simulink model "Model0"  (R2022b)
settings: Solver=VariableStepAuto  StartTime=0.0  StopTime=10.0  RelTol=1e-3
undefined symbols (not defined in the file or in its folder): commpassbandmodParams, qam_params
libraries: hdlsllib x14, dspsrcs4 x9, commfilt2 x8, commdigbbndam3 x8
settings Model: Creator=Ceribro  LastModifiedBy=Ceribro

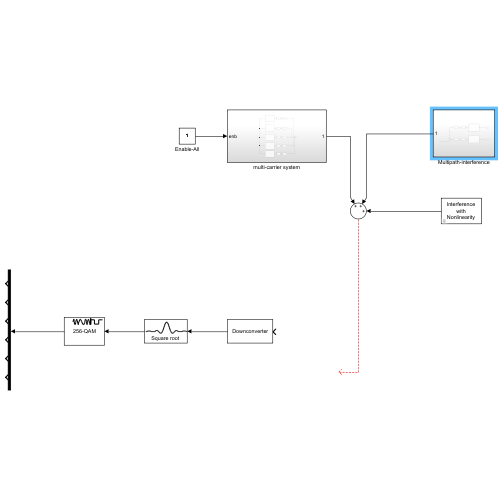
[thumbnail: Simulink's stored preview of the top-level diagram]
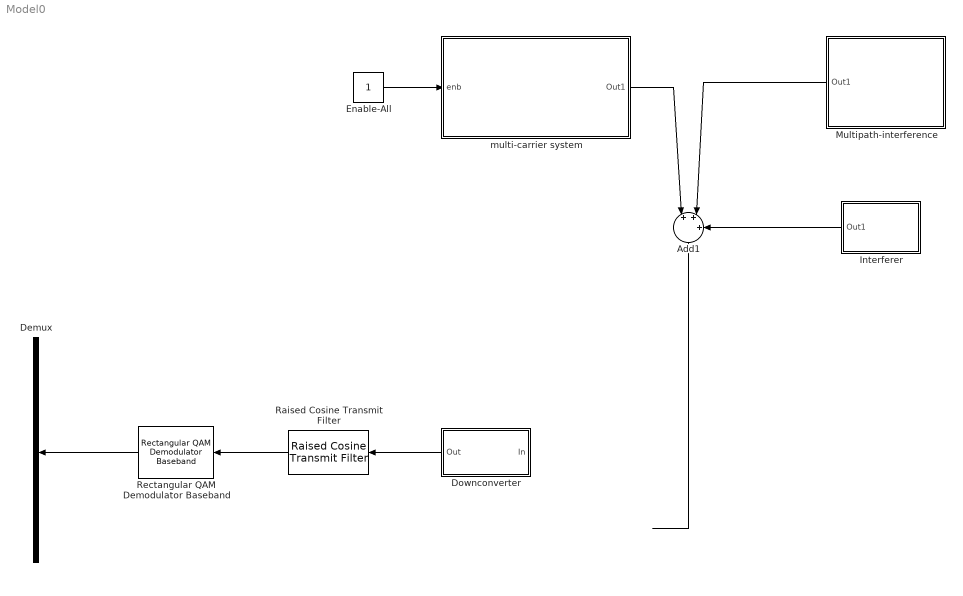
== system Model0 ==
  Add1 : Sum  Inputs=|+++
  Demux : Demux  Outputs=6
  Downconverter : Subsystem
      mask Display: disp('Downconverter')
  Enable-All : Constant  OutDataTypeStr=boolean
  Interferer : Subsystem  mask(Interference){nonlinOrder=3}
      mask prompts: nonlinOrder "Order of nonlinearity:"
      mask help: Generate out-of-band interference. Optionally process the interference with a third-order nonlinearity that creates an in-band harmonic.
      mask init:
      | if nonlinOrder == 1
      |     icontext = 'Interference\nwithout\nNonlinearity';
      | elseif nonlinOrder == 3
      |     icontext = 'Interference\nwith\nNonlinearity';
      | end
      mask Display: disp(icontext)
  Multipath-interference : Subsystem
  Raised Cosine Transmit Filter : commfilt2/Raised Cosine Transmit Filter  filtType=Square root  R=0.2  filtSpan=8  N=8  filterGain=1  InputProcessing=Columns as channels (frame based)  RateOptions=Enforce single-rate processing  framing=Mute  checkCoeff=off  variableName=rcTxFilt1  checkGain=Normalized  sampMode=Mute  saveAsFlag=0  currentFiltSpan=2*(4)  D=4  launchFVT=off  roundingMode=Floor  overflowMode=off  coeffDataTypeStr=Inherit: Same word length as input  coeffMin=[]  coeffMax=[]  coeffLastDataTypeStr=Inherit: Same word length as input  outputDataTypeStr=Inherit: Same as accumulator  outputMin=[]  outputMax=[]  outputLastDataTypeStr=Inherit: Same as accumulator
  Rectangular QAM Demodulator Baseband : commdigbbndam3/Rectangular QAM Demodulator Baseband  M=256  OutType=Integer  DecType=Hard decision  VarSource=Dialog  Variance=1  Dec=Gray  Mapping=[0:15]  PowType=Min. distance between symbols  MinDist=2  AvgPow=1  PeakPow=1  Ph=0  outDtype1=Inherit via internal rule  outDtype2=Inherit via internal rule  derotateFactorWordLen=16  derotateFactorDataTypeStr=Inherit: Same word length as input  derotateFactorLastDataTypeStr=Inherit: Same word length as input  denormFactorWordLen=16  denormFactorDataTypeStr=Inherit: Same word length as input  denormFactorLastDataTypeStr=Inherit: Same word length as input  prodOutWordLen=32  prodOutOverflowMode=Wrap  prodOutRoundingMode=Floor  prodOutOvFlMode=off  prodOutOvFlModeLastStrValue=off  sumWordLen=32
      settings: LibrarySourceBlock=|
      | commhdldigbbndam/Rectangular QAM
      | Demodulator
      | Baseband
  multi-carrier system : Subsystem
  wires:
  Enable-All/1 -> multi-carrier system/1(enb)
  multi-carrier system/1(Out1) -> Add1/1
  Multipath-interference/1(Out1) -> Add1/2
  Interferer/1(Out1) -> Add1/3
  Add1/1 -> ?
  Downconverter/1(Out) -> Raised Cosine Transmit Filter/1
  Raised Cosine Transmit Filter/1 -> Rectangular QAM Demodulator Baseband/1
  Rectangular QAM Demodulator Baseband/1 -> Demux/1

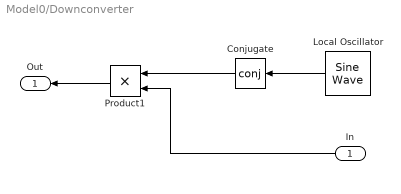
== system Model0/Downconverter ==
  In : Inport
  Conjugate : Math  Operator=conj  SignedPower=on
  Local Oscillator : dspsrcs4/Sine Wave  Amplitude=1  Frequency=commpassbandmodParams.Fc  Phase=0  SampleMode=Discrete  OutComplex=Complex  CompMethod=Trigonometric fcn  TableSize=Speed  SampleTime=(1e-6) /8  SamplesPerFrame=800  ResetState=Restart at time zero  OutputFrames=off  dataType=double  wordLen=16  udDataType=sfix(16)  fracBitsMode=Best precision  numFracBits=15  OutDataTypeStr=double  LastOutDataTypeStr=double
  Product1 : Product  RndMeth=Zero
  Out : Outport  VectorParamsAs1DForOutWhenUnconnected=off
  wires:
  Conjugate/1 -> Product1/1
  Product1/1 -> Out/1
  In/1 -> Product1/2
  Local Oscillator/1 -> Conjugate/1

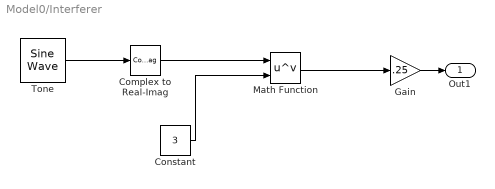
== system Model0/Interferer ==
  Complex to Real-Imag : ComplexToRealImag  Output=Real
  Constant : Constant  Value=3
  Gain : Gain  Gain=.25
  Math Function : Math  Operator=pow  SignedPower=on
  "Tone " : dspsrcs4/Sine Wave  Amplitude=1  Frequency=8.8333e+05  Phase=0  SampleMode=Discrete  OutComplex=Complex  CompMethod=Trigonometric fcn  TableSize=Speed  SampleTime=(1e-6) /8  SamplesPerFrame=800  ResetState=Restart at time zero  OutputFrames=off  dataType=double  wordLen=16  udDataType=sfix(16)  fracBitsMode=Best precision  numFracBits=15  OutDataTypeStr=double  LastOutDataTypeStr=double
  Out1 : Outport  VectorParamsAs1DForOutWhenUnconnected=off
  wires:
  Complex to Real-Imag/1 -> Math Function/1
  Constant/1 -> Math Function/2
  "Tone "/1 -> Complex to Real-Imag/1
  Math Function/1 -> Gain/1
  Gain/1 -> Out1/1

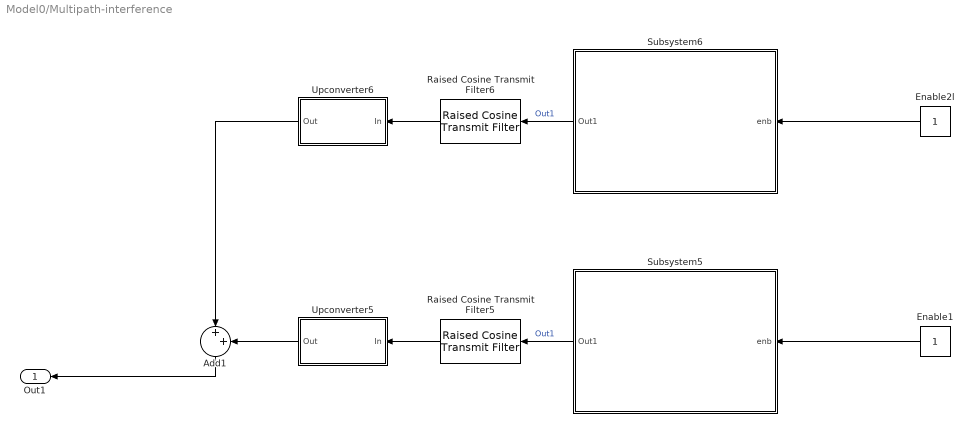
== system Model0/Multipath-interference ==
  Add1 : Sum  Inputs=|++
  Enable1 : Constant  OutDataTypeStr=boolean
  Enable2l : Constant  OutDataTypeStr=boolean
  Raised Cosine Transmit Filter5 : commfilt2/Raised Cosine Transmit Filter  filtType=Square root  R=0.2  filtSpan=8  N=8  filterGain=1  InputProcessing=Columns as channels (frame based)  RateOptions=Enforce single-rate processing  framing=Mute  checkCoeff=off  variableName=rcTxFilt5  checkGain=Normalized  sampMode=Mute  saveAsFlag=0  currentFiltSpan=2*(4)  D=4  launchFVT=off  roundingMode=Floor  overflowMode=off  coeffDataTypeStr=Inherit: Same word length as input  coeffMin=[]  coeffMax=[]  coeffLastDataTypeStr=Inherit: Same word length as input  outputDataTypeStr=Inherit: Same as accumulator  outputMin=[]  outputMax=[]  outputLastDataTypeStr=Inherit: Same as accumulator
  Raised Cosine Transmit Filter6 : commfilt2/Raised Cosine Transmit Filter  filtType=Square root  R=0.2  filtSpan=8  N=8  filterGain=1  InputProcessing=Columns as channels (frame based)  RateOptions=Enforce single-rate processing  framing=Mute  checkCoeff=off  variableName=rcTxFilt6  checkGain=Normalized  sampMode=Mute  saveAsFlag=0  currentFiltSpan=2*(4)  D=4  launchFVT=off  roundingMode=Floor  overflowMode=off  coeffDataTypeStr=Inherit: Same word length as input  coeffMin=[]  coeffMax=[]  coeffLastDataTypeStr=Inherit: Same word length as input  outputDataTypeStr=Inherit: Same as accumulator  outputMin=[]  outputMax=[]  outputLastDataTypeStr=Inherit: Same as accumulator
  Subsystem5 : Subsystem
  Subsystem6 : Subsystem
  Upconverter5 : Subsystem
      mask Display: disp('Upconverter')
  Upconverter6 : Subsystem
      mask Display: disp('Upconverter')
  Out1 : Outport
  wires:
  Upconverter5/1(Out) -> Add1/2
  Raised Cosine Transmit Filter5/1 -> Upconverter5/1(In)
  Raised Cosine Transmit Filter6/1 -> Upconverter6/1(In)
  Subsystem6/1(Out1) -> Raised Cosine Transmit Filter6/1  "Out1"
  Enable1/1 -> Subsystem5/1(enb)
  Subsystem5/1(Out1) -> Raised Cosine Transmit Filter5/1  "Out1"
  Enable2l/1 -> Subsystem6/1(enb)
  Upconverter6/1(Out) -> Add1/1
  Add1/1 -> Out1/1

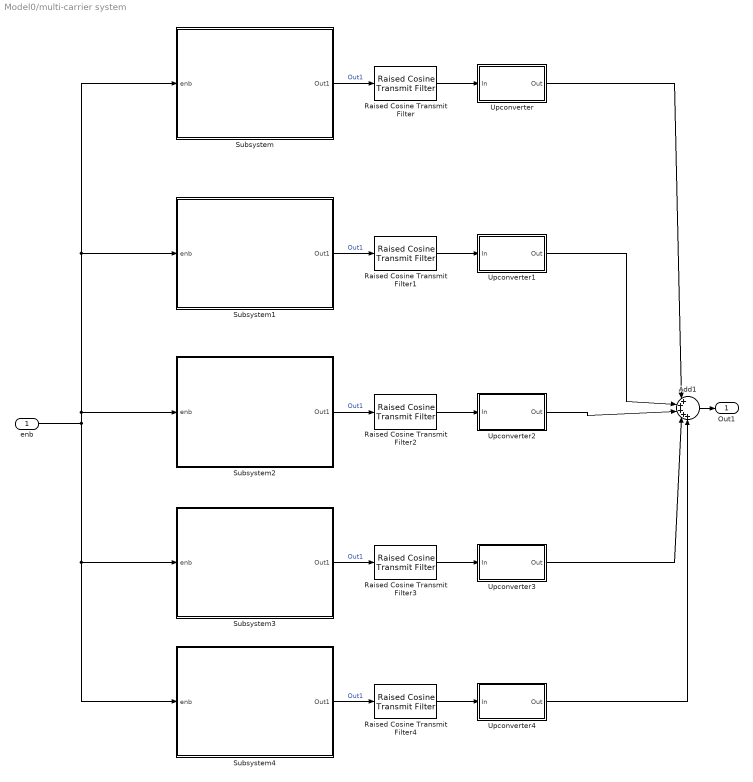
== system Model0/multi-carrier system ==
  enb : Inport
  Add1 : Sum  Inputs=|+++++
  Raised Cosine Transmit Filter : commfilt2/Raised Cosine Transmit Filter  filtType=Square root  R=0.2  filtSpan=8  N=8  filterGain=1  InputProcessing=Columns as channels (frame based)  RateOptions=Enforce single-rate processing  framing=Mute  checkCoeff=off  variableName=rcTxFilt1  checkGain=Normalized  sampMode=Mute  saveAsFlag=0  currentFiltSpan=2*(4)  D=4  launchFVT=off  roundingMode=Floor  overflowMode=off  coeffDataTypeStr=Inherit: Same word length as input  coeffMin=[]  coeffMax=[]  coeffLastDataTypeStr=Inherit: Same word length as input  outputDataTypeStr=Inherit: Same as accumulator  outputMin=[]  outputMax=[]  outputLastDataTypeStr=Inherit: Same as accumulator
  Raised Cosine Transmit Filter1 : commfilt2/Raised Cosine Transmit Filter  filtType=Square root  R=0.2  filtSpan=8  N=8  filterGain=1  InputProcessing=Columns as channels (frame based)  RateOptions=Enforce single-rate processing  framing=Mute  checkCoeff=off  variableName=rcTxFilt1  checkGain=Normalized  sampMode=Mute  saveAsFlag=0  currentFiltSpan=2*(4)  D=4  launchFVT=off  roundingMode=Floor  overflowMode=off  coeffDataTypeStr=Inherit: Same word length as input  coeffMin=[]  coeffMax=[]  coeffLastDataTypeStr=Inherit: Same word length as input  outputDataTypeStr=Inherit: Same as accumulator  outputMin=[]  outputMax=[]  outputLastDataTypeStr=Inherit: Same as accumulator
  Raised Cosine Transmit Filter2 : commfilt2/Raised Cosine Transmit Filter  filtType=Square root  R=0.2  filtSpan=8  N=8  filterGain=1  InputProcessing=Columns as channels (frame based)  RateOptions=Enforce single-rate processing  framing=Mute  checkCoeff=off  variableName=rcTxFilt2  checkGain=Normalized  sampMode=Mute  saveAsFlag=0  currentFiltSpan=2*(4)  D=4  launchFVT=off  roundingMode=Floor  overflowMode=off  coeffDataTypeStr=Inherit: Same word length as input  coeffMin=[]  coeffMax=[]  coeffLastDataTypeStr=Inherit: Same word length as input  outputDataTypeStr=Inherit: Same as accumulator  outputMin=[]  outputMax=[]  outputLastDataTypeStr=Inherit: Same as accumulator
  Raised Cosine Transmit Filter3 : commfilt2/Raised Cosine Transmit Filter  filtType=Square root  R=0.2  filtSpan=8  N=8  filterGain=1  InputProcessing=Columns as channels (frame based)  RateOptions=Enforce single-rate processing  framing=Mute  checkCoeff=off  variableName=rcTxFilt3  checkGain=Normalized  sampMode=Mute  saveAsFlag=0  currentFiltSpan=2*(4)  D=4  launchFVT=off  roundingMode=Floor  overflowMode=off  coeffDataTypeStr=Inherit: Same word length as input  coeffMin=[]  coeffMax=[]  coeffLastDataTypeStr=Inherit: Same word length as input  outputDataTypeStr=Inherit: Same as accumulator  outputMin=[]  outputMax=[]  outputLastDataTypeStr=Inherit: Same as accumulator
  Raised Cosine Transmit Filter4 : commfilt2/Raised Cosine Transmit Filter  filtType=Square root  R=0.2  filtSpan=8  N=8  filterGain=1  InputProcessing=Columns as channels (frame based)  RateOptions=Enforce single-rate processing  framing=Mute  checkCoeff=off  variableName=rcTxFilt4  checkGain=Normalized  sampMode=Mute  saveAsFlag=0  currentFiltSpan=2*(4)  D=4  launchFVT=off  roundingMode=Floor  overflowMode=off  coeffDataTypeStr=Inherit: Same word length as input  coeffMin=[]  coeffMax=[]  coeffLastDataTypeStr=Inherit: Same word length as input  outputDataTypeStr=Inherit: Same as accumulator  outputMin=[]  outputMax=[]  outputLastDataTypeStr=Inherit: Same as accumulator
  Subsystem : Subsystem
  Subsystem1 : Subsystem
  Subsystem2 : Subsystem
  Subsystem3 : Subsystem
  Subsystem4 : Subsystem
  Upconverter : Subsystem
      mask Display: disp('Upconverter')
  Upconverter1 : Subsystem
      mask Display: disp('Upconverter')
  Upconverter2 : Subsystem
      mask Display: disp('Upconverter')
  Upconverter3 : Subsystem
      mask Display: disp('Upconverter')
  Upconverter4 : Subsystem
      mask Display: disp('Upconverter')
  Out1 : Outport
  wires:
  enb/1 -> Subsystem/1(enb), Subsystem1/1(enb), Subsystem2/1(enb), Subsystem4/1(enb), Subsystem3/1(enb)
  Upconverter3/1(Out) -> Add1/4
  Subsystem1/1(Out1) -> Raised Cosine Transmit Filter1/1  "Out1"
  Raised Cosine Transmit Filter/1 -> Upconverter/1(In)
  Upconverter/1(Out) -> Add1/1
  Upconverter2/1(Out) -> Add1/3
  Upconverter1/1(Out) -> Add1/2
  Raised Cosine Transmit Filter1/1 -> Upconverter1/1(In)
  Raised Cosine Transmit Filter3/1 -> Upconverter3/1(In)
  Upconverter4/1(Out) -> Add1/5
  Raised Cosine Transmit Filter2/1 -> Upconverter2/1(In)
  Add1/1 -> Out1/1
  Subsystem2/1(Out1) -> Raised Cosine Transmit Filter2/1  "Out1"
  Subsystem3/1(Out1) -> Raised Cosine Transmit Filter3/1  "Out1"
  Subsystem/1(Out1) -> Raised Cosine Transmit Filter/1  "Out1"
  Raised Cosine Transmit Filter4/1 -> Upconverter4/1(In)
  Subsystem4/1(Out1) -> Raised Cosine Transmit Filter4/1  "Out1"

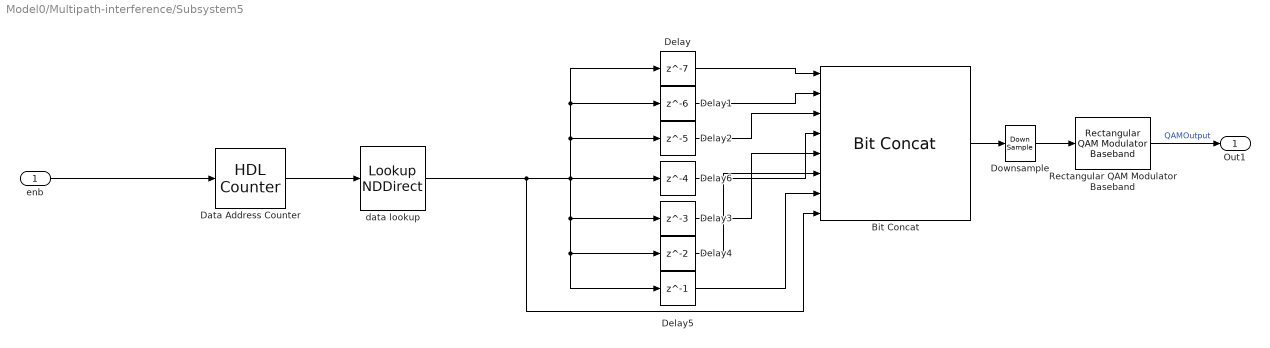
== system Model0/Multipath-interference/Subsystem5 ==
  enb : Inport
  Bit Concat : hdlsllib/Logic and Bit Operations/Bit Concat  numInputs=8
  Data Address Counter : hdlsllib/Sources/HDL Counter  CountType=Count limited  CountInit=0  CountStep=1  CountMax=qam_params.total_data_bits-1  CountFromType=Initial value  CountFrom=0  CountResetPort=off  CountLoadPort=off  CountEnbPort=on  CountDirPort=off  CountHitOutputPort=off  CountDataType=Unsigned  CountWordLen=16  CountFracLen=0  CountSampTime=1
  Delay : Delay  DelayLength=7  InitialCondition=0
  Delay1 : Delay  DelayLength=6  InitialCondition=0
  Delay2 : Delay  DelayLength=5  InitialCondition=0
  Delay3 : Delay  DelayLength=3  InitialCondition=0
  Delay4 : Delay  InitialCondition=0
  Delay5 : Delay  DelayLength=1  InitialCondition=0
  Delay6 : Delay  DelayLength=4  InitialCondition=0
  Downsample : DownSample  N=8  RateOptions=Allow multirate processing
  Rectangular QAM Modulator Baseband : commdigbbndam3/Rectangular QAM Modulator Baseband  M=256  InType=Integer  Enc=Gray  Mapping=[0:15]  PowType=Min. distance between symbols  MinDist=2  AvgPow=1  PeakPow=1  Ph=0  outDtype=double  outWordLen=16  outUDDataType=sfix(16)  outFracLenMode=Best precision  outFracLen=15  outDataTypeStr=double  outLastDataTypeStr=double
      settings: LibrarySourceBlock=|
      | commhdldigbbndam/Rectangular QAM
      | Modulator
      | Baseband
  data lookup : LookupNDDirect  NumberOfTableDimensions=1  Table=qam_params.tx_data_bits  DiagnosticForOutOfRangeInput=Error  SampleTime=1/qam_params.bitRate  TableDataTypeStr=boolean
  Out1 : Outport
  wires:
  data lookup/1 -> Bit Concat/8, Delay5/1, Delay4/1, Delay3/1, Delay6/1, Delay/1, Delay1/1, Delay2/1
  Delay5/1 -> Bit Concat/7
  Delay2/1 -> Bit Concat/3
  Delay3/1 -> Bit Concat/5
  Data Address Counter/1 -> data lookup/1
  Delay1/1 -> Bit Concat/2
  Bit Concat/1 -> Downsample/1
  Delay6/1 -> Bit Concat/4
  Delay/1 -> Bit Concat/1
  enb/1 -> Data Address Counter/1
  Delay4/1 -> Bit Concat/6
  Rectangular QAM Modulator Baseband/1 -> Out1/1  "QAMOutput"
  Downsample/1 -> Rectangular QAM Modulator Baseband/1

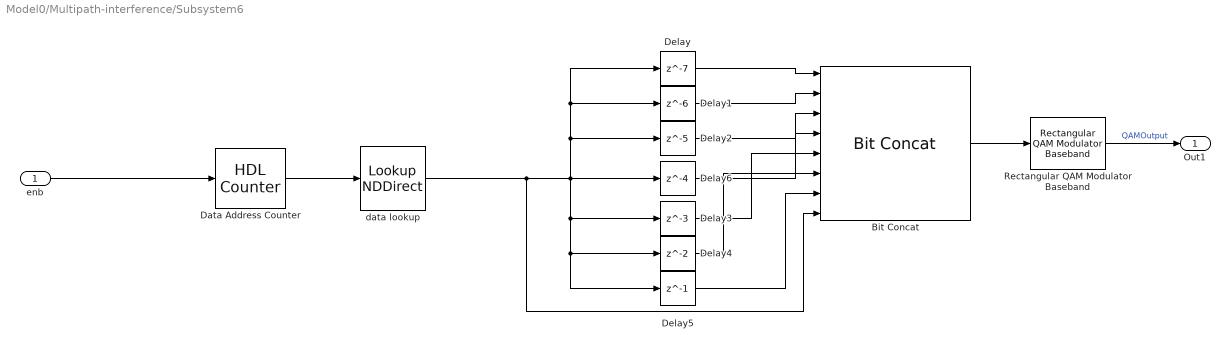
== system Model0/Multipath-interference/Subsystem6 ==
  enb : Inport
  Bit Concat : hdlsllib/Logic and Bit Operations/Bit Concat  numInputs=8
  Data Address Counter : hdlsllib/Sources/HDL Counter  CountType=Count limited  CountInit=0  CountStep=1  CountMax=qam_params.total_data_bits-1  CountFromType=Initial value  CountFrom=0  CountResetPort=off  CountLoadPort=off  CountEnbPort=on  CountDirPort=off  CountHitOutputPort=off  CountDataType=Signed  CountWordLen=16  CountFracLen=0  CountSampTime=1
  Delay : Delay  DelayLength=7  InitialCondition=0
  Delay1 : Delay  DelayLength=6  InitialCondition=0
  Delay2 : Delay  DelayLength=5  InitialCondition=0
  Delay3 : Delay  DelayLength=3  InitialCondition=0
  Delay4 : Delay  InitialCondition=0
  Delay5 : Delay  DelayLength=1  InitialCondition=0
  Delay6 : Delay  DelayLength=4  InitialCondition=0
  Rectangular QAM Modulator Baseband : commdigbbndam3/Rectangular QAM Modulator Baseband  M=256  InType=Integer  Enc=Gray  Mapping=[0:15]  PowType=Min. distance between symbols  MinDist=2  AvgPow=1  PeakPow=1  Ph=0  outDtype=double  outWordLen=16  outUDDataType=sfix(16)  outFracLenMode=Best precision  outFracLen=15  outDataTypeStr=double  outLastDataTypeStr=double
      settings: LibrarySourceBlock=|
      | commhdldigbbndam/Rectangular QAM
      | Modulator
      | Baseband
  data lookup : LookupNDDirect  NumberOfTableDimensions=1  Table=qam_params.tx_data_bits  DiagnosticForOutOfRangeInput=Error  SampleTime=1/qam_params.bitRate  TableDataTypeStr=boolean
  Out1 : Outport
  wires:
  data lookup/1 -> Bit Concat/8, Delay5/1, Delay4/1, Delay3/1, Delay6/1, Delay/1, Delay1/1, Delay2/1
  Delay5/1 -> Bit Concat/7
  Delay2/1 -> Bit Concat/3
  Delay3/1 -> Bit Concat/5
  Data Address Counter/1 -> data lookup/1
  Delay1/1 -> Bit Concat/2
  Bit Concat/1 -> Rectangular QAM Modulator Baseband/1
  Delay6/1 -> Bit Concat/4
  Delay/1 -> Bit Concat/1
  enb/1 -> Data Address Counter/1
  Delay4/1 -> Bit Concat/6
  Rectangular QAM Modulator Baseband/1 -> Out1/1  "QAMOutput"

== system Model0/Multipath-interference/Upconverter5 ==
  In : Inport
  Complex to Real-Imag : ComplexToRealImag  Output=Real
  Local Oscillator : dspsrcs4/Sine Wave  Amplitude=1  Frequency=200e6  Phase=0  SampleMode=Discrete  OutComplex=Complex  CompMethod=Trigonometric fcn  TableSize=Speed  SampleTime=(1e-6) /8  SamplesPerFrame=8  ResetState=Restart at time zero  OutputFrames=off  dataType=double  wordLen=16  udDataType=sfix(16)  fracBitsMode=Best precision  numFracBits=15  OutDataTypeStr=double  LastOutDataTypeStr=double
  Product : Product  RndMeth=Zero
  Out : Outport  VectorParamsAs1DForOutWhenUnconnected=off
  wires:
  Complex to Real-Imag/1 -> Out/1
  Product/1 -> Complex to Real-Imag/1
  Local Oscillator/1 -> Product/2
  In/1 -> Product/1

== system Model0/Multipath-interference/Upconverter6 ==
  In : Inport
  Complex to Real-Imag : ComplexToRealImag  Output=Real
  Local Oscillator : dspsrcs4/Sine Wave  Amplitude=1  Frequency=400e6  Phase=0  SampleMode=Discrete  OutComplex=Complex  CompMethod=Trigonometric fcn  TableSize=Speed  SampleTime=(1e-6) /8  SamplesPerFrame=8  ResetState=Restart at time zero  OutputFrames=off  dataType=double  wordLen=16  udDataType=sfix(16)  fracBitsMode=Best precision  numFracBits=15  OutDataTypeStr=double  LastOutDataTypeStr=double
  Product : Product  RndMeth=Zero
  Out : Outport  VectorParamsAs1DForOutWhenUnconnected=off
  wires:
  Complex to Real-Imag/1 -> Out/1
  Product/1 -> Complex to Real-Imag/1
  Local Oscillator/1 -> Product/2
  In/1 -> Product/1

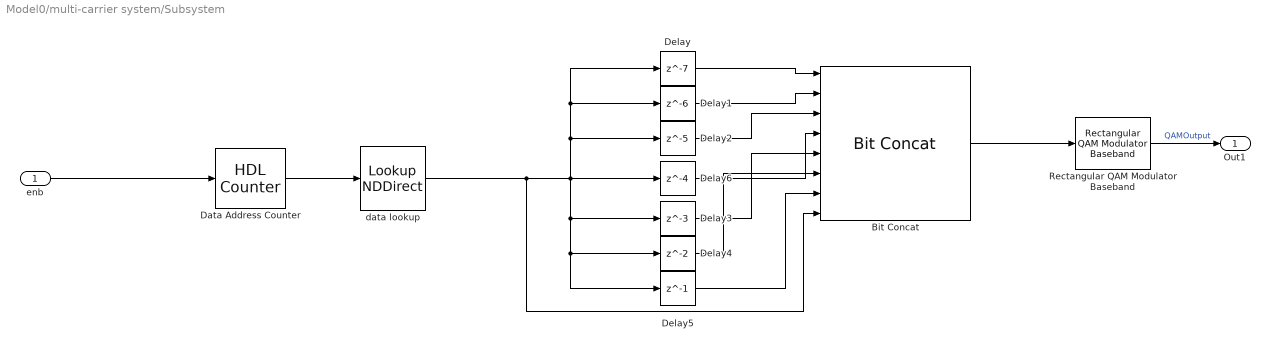
== system Model0/multi-carrier system/Subsystem ==
  enb : Inport
  Bit Concat : hdlsllib/Logic and Bit Operations/Bit Concat  numInputs=8
  Data Address Counter : hdlsllib/Sources/HDL Counter  CountType=Count limited  CountInit=0  CountStep=1  CountMax=qam_params.total_data_bits-1  CountFromType=Initial value  CountFrom=0  CountResetPort=off  CountLoadPort=off  CountEnbPort=on  CountDirPort=off  CountHitOutputPort=off  CountDataType=Unsigned  CountWordLen=16  CountFracLen=0  CountSampTime=1
  Delay : Delay  DelayLength=7  InitialCondition=0
  Delay1 : Delay  DelayLength=6  InitialCondition=0
  Delay2 : Delay  DelayLength=5  InitialCondition=0
  Delay3 : Delay  DelayLength=3  InitialCondition=0
  Delay4 : Delay  InitialCondition=0
  Delay5 : Delay  DelayLength=1  InitialCondition=0
  Delay6 : Delay  DelayLength=4  InitialCondition=0
  Rectangular QAM Modulator Baseband : commdigbbndam3/Rectangular QAM Modulator Baseband  M=256  InType=Integer  Enc=Gray  Mapping=[0:15]  PowType=Min. distance between symbols  MinDist=2  AvgPow=1  PeakPow=1  Ph=0  outDtype=double  outWordLen=16  outUDDataType=sfix(16)  outFracLenMode=Best precision  outFracLen=15  outDataTypeStr=double  outLastDataTypeStr=double
      settings: LibrarySourceBlock=|
      | commhdldigbbndam/Rectangular QAM
      | Modulator
      | Baseband
  data lookup : LookupNDDirect  NumberOfTableDimensions=1  Table=qam_params.tx_data_bits  DiagnosticForOutOfRangeInput=Error  SampleTime=1/qam_params.bitRate  TableDataTypeStr=boolean
  Out1 : Outport
  wires:
  data lookup/1 -> Bit Concat/8, Delay5/1, Delay4/1, Delay3/1, Delay6/1, Delay/1, Delay1/1, Delay2/1
  Delay5/1 -> Bit Concat/7
  Delay2/1 -> Bit Concat/3
  Delay3/1 -> Bit Concat/5
  Data Address Counter/1 -> data lookup/1
  Delay1/1 -> Bit Concat/2
  Delay6/1 -> Bit Concat/4
  Delay/1 -> Bit Concat/1
  enb/1 -> Data Address Counter/1
  Delay4/1 -> Bit Concat/6
  Rectangular QAM Modulator Baseband/1 -> Out1/1  "QAMOutput"
  Bit Concat/1 -> Rectangular QAM Modulator Baseband/1

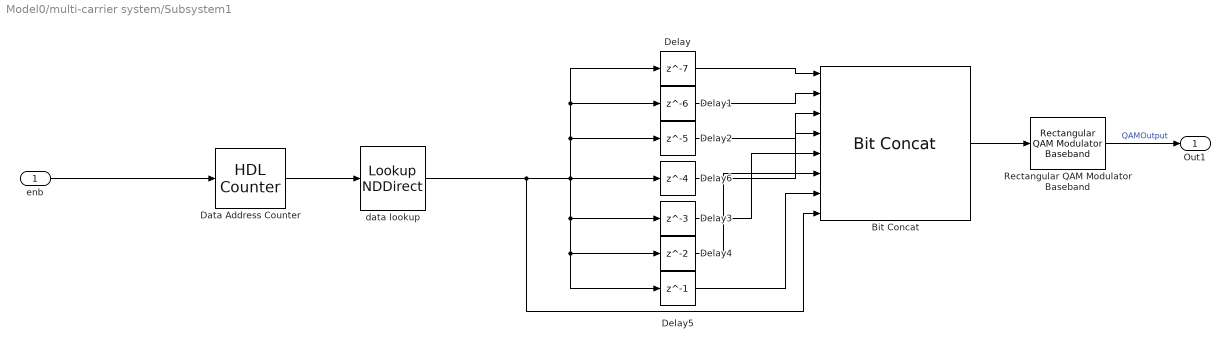
== system Model0/multi-carrier system/Subsystem1 ==
  enb : Inport
  Bit Concat : hdlsllib/Logic and Bit Operations/Bit Concat  numInputs=8
  Data Address Counter : hdlsllib/Sources/HDL Counter  CountType=Count limited  CountInit=0  CountStep=1  CountMax=qam_params.total_data_bits-1  CountFromType=Initial value  CountFrom=0  CountResetPort=off  CountLoadPort=off  CountEnbPort=on  CountDirPort=off  CountHitOutputPort=off  CountDataType=Unsigned  CountWordLen=16  CountFracLen=0  CountSampTime=1
  Delay : Delay  DelayLength=7  InitialCondition=0
  Delay1 : Delay  DelayLength=6  InitialCondition=0
  Delay2 : Delay  DelayLength=5  InitialCondition=0
  Delay3 : Delay  DelayLength=3  InitialCondition=0
  Delay4 : Delay  InitialCondition=0
  Delay5 : Delay  DelayLength=1  InitialCondition=0
  Delay6 : Delay  DelayLength=4  InitialCondition=0
  Rectangular QAM Modulator Baseband : commdigbbndam3/Rectangular QAM Modulator Baseband  M=256  InType=Integer  Enc=Gray  Mapping=[0:15]  PowType=Min. distance between symbols  MinDist=2  AvgPow=1  PeakPow=1  Ph=0  outDtype=double  outWordLen=16  outUDDataType=sfix(16)  outFracLenMode=Best precision  outFracLen=15  outDataTypeStr=double  outLastDataTypeStr=double
      settings: LibrarySourceBlock=|
      | commhdldigbbndam/Rectangular QAM
      | Modulator
      | Baseband
  data lookup : LookupNDDirect  NumberOfTableDimensions=1  Table=qam_params.tx_data_bits  DiagnosticForOutOfRangeInput=Error  SampleTime=1/qam_params.bitRate  TableDataTypeStr=boolean
  Out1 : Outport
  wires:
  data lookup/1 -> Bit Concat/8, Delay5/1, Delay4/1, Delay3/1, Delay6/1, Delay/1, Delay1/1, Delay2/1
  Delay5/1 -> Bit Concat/7
  Delay2/1 -> Bit Concat/3
  Delay3/1 -> Bit Concat/5
  Data Address Counter/1 -> data lookup/1
  Delay1/1 -> Bit Concat/2
  Bit Concat/1 -> Rectangular QAM Modulator Baseband/1
  Delay6/1 -> Bit Concat/4
  Delay/1 -> Bit Concat/1
  enb/1 -> Data Address Counter/1
  Delay4/1 -> Bit Concat/6
  Rectangular QAM Modulator Baseband/1 -> Out1/1  "QAMOutput"

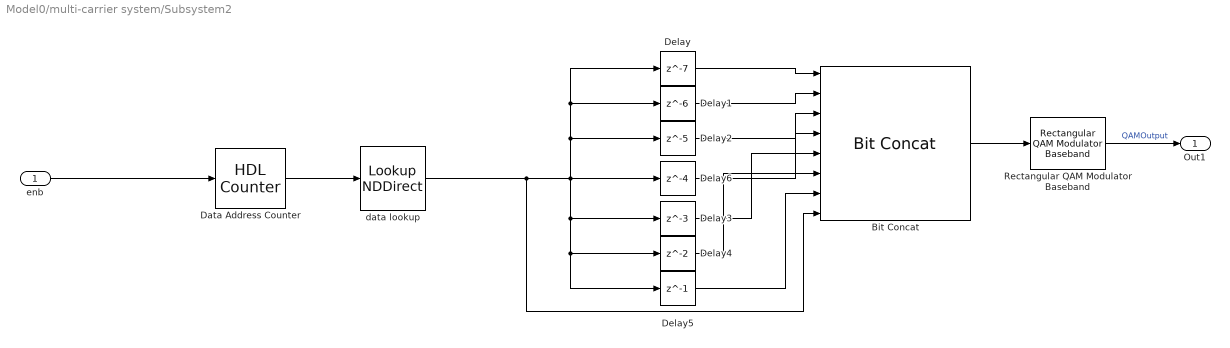
== system Model0/multi-carrier system/Subsystem2 ==
  enb : Inport
  Bit Concat : hdlsllib/Logic and Bit Operations/Bit Concat  numInputs=8
  Data Address Counter : hdlsllib/Sources/HDL Counter  CountType=Count limited  CountInit=0  CountStep=1  CountMax=qam_params.total_data_bits-1  CountFromType=Initial value  CountFrom=0  CountResetPort=off  CountLoadPort=off  CountEnbPort=on  CountDirPort=off  CountHitOutputPort=off  CountDataType=Unsigned  CountWordLen=16  CountFracLen=0  CountSampTime=1
  Delay : Delay  DelayLength=7  InitialCondition=0
  Delay1 : Delay  DelayLength=6  InitialCondition=0
  Delay2 : Delay  DelayLength=5  InitialCondition=0
  Delay3 : Delay  DelayLength=3  InitialCondition=0
  Delay4 : Delay  InitialCondition=0
  Delay5 : Delay  DelayLength=1  InitialCondition=0
  Delay6 : Delay  DelayLength=4  InitialCondition=0
  Rectangular QAM Modulator Baseband : commdigbbndam3/Rectangular QAM Modulator Baseband  M=256  InType=Integer  Enc=Gray  Mapping=[0:15]  PowType=Min. distance between symbols  MinDist=2  AvgPow=1  PeakPow=1  Ph=0  outDtype=double  outWordLen=16  outUDDataType=sfix(16)  outFracLenMode=Best precision  outFracLen=15  outDataTypeStr=double  outLastDataTypeStr=double
      settings: LibrarySourceBlock=|
      | commhdldigbbndam/Rectangular QAM
      | Modulator
      | Baseband
  data lookup : LookupNDDirect  NumberOfTableDimensions=1  Table=qam_params.tx_data_bits  DiagnosticForOutOfRangeInput=Error  SampleTime=1/qam_params.bitRate  TableDataTypeStr=boolean
  Out1 : Outport
  wires:
  data lookup/1 -> Bit Concat/8, Delay5/1, Delay4/1, Delay3/1, Delay6/1, Delay/1, Delay1/1, Delay2/1
  Delay5/1 -> Bit Concat/7
  Delay2/1 -> Bit Concat/3
  Delay3/1 -> Bit Concat/5
  Data Address Counter/1 -> data lookup/1
  Delay1/1 -> Bit Concat/2
  Bit Concat/1 -> Rectangular QAM Modulator Baseband/1
  Delay6/1 -> Bit Concat/4
  Delay/1 -> Bit Concat/1
  enb/1 -> Data Address Counter/1
  Delay4/1 -> Bit Concat/6
  Rectangular QAM Modulator Baseband/1 -> Out1/1  "QAMOutput"

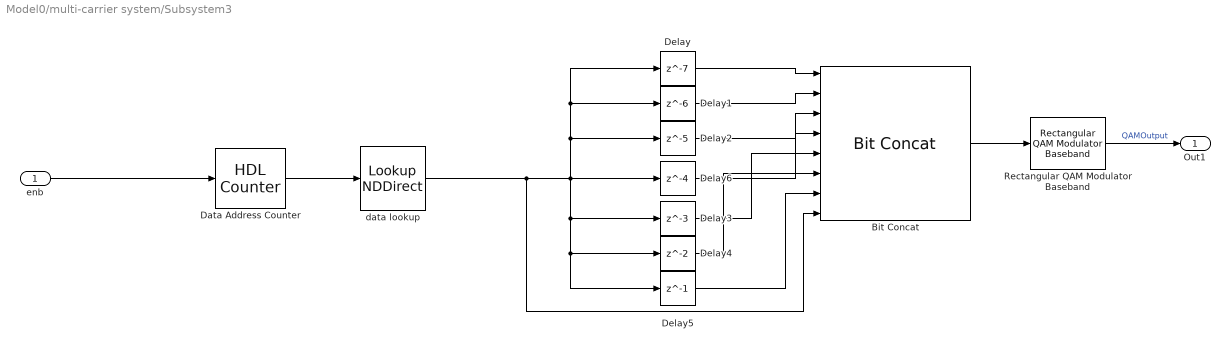
== system Model0/multi-carrier system/Subsystem3 ==
  enb : Inport
  Bit Concat : hdlsllib/Logic and Bit Operations/Bit Concat  numInputs=8
  Data Address Counter : hdlsllib/Sources/HDL Counter  CountType=Count limited  CountInit=0  CountStep=1  CountMax=qam_params.total_data_bits-1  CountFromType=Initial value  CountFrom=0  CountResetPort=off  CountLoadPort=off  CountEnbPort=on  CountDirPort=off  CountHitOutputPort=off  CountDataType=Unsigned  CountWordLen=16  CountFracLen=0  CountSampTime=1
  Delay : Delay  DelayLength=7  InitialCondition=0
  Delay1 : Delay  DelayLength=6  InitialCondition=0
  Delay2 : Delay  DelayLength=5  InitialCondition=0
  Delay3 : Delay  DelayLength=3  InitialCondition=0
  Delay4 : Delay  InitialCondition=0
  Delay5 : Delay  DelayLength=1  InitialCondition=0
  Delay6 : Delay  DelayLength=4  InitialCondition=0
  Rectangular QAM Modulator Baseband : commdigbbndam3/Rectangular QAM Modulator Baseband  M=256  InType=Integer  Enc=Gray  Mapping=[0:15]  PowType=Min. distance between symbols  MinDist=2  AvgPow=1  PeakPow=1  Ph=0  outDtype=double  outWordLen=16  outUDDataType=sfix(16)  outFracLenMode=Best precision  outFracLen=15  outDataTypeStr=double  outLastDataTypeStr=double
      settings: LibrarySourceBlock=|
      | commhdldigbbndam/Rectangular QAM
      | Modulator
      | Baseband
  data lookup : LookupNDDirect  NumberOfTableDimensions=1  Table=qam_params.tx_data_bits  DiagnosticForOutOfRangeInput=Error  SampleTime=1/qam_params.bitRate  TableDataTypeStr=boolean
  Out1 : Outport
  wires:
  data lookup/1 -> Bit Concat/8, Delay5/1, Delay4/1, Delay3/1, Delay6/1, Delay/1, Delay1/1, Delay2/1
  Delay5/1 -> Bit Concat/7
  Delay2/1 -> Bit Concat/3
  Delay3/1 -> Bit Concat/5
  Data Address Counter/1 -> data lookup/1
  Delay1/1 -> Bit Concat/2
  Bit Concat/1 -> Rectangular QAM Modulator Baseband/1
  Delay6/1 -> Bit Concat/4
  Delay/1 -> Bit Concat/1
  enb/1 -> Data Address Counter/1
  Delay4/1 -> Bit Concat/6
  Rectangular QAM Modulator Baseband/1 -> Out1/1  "QAMOutput"

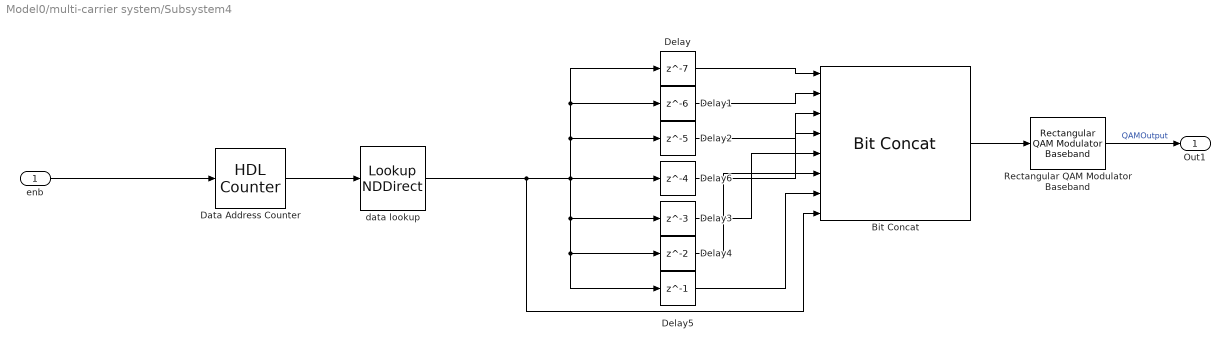
== system Model0/multi-carrier system/Subsystem4 ==
  enb : Inport
  Bit Concat : hdlsllib/Logic and Bit Operations/Bit Concat  numInputs=8
  Data Address Counter : hdlsllib/Sources/HDL Counter  CountType=Count limited  CountInit=0  CountStep=1  CountMax=qam_params.total_data_bits-1  CountFromType=Initial value  CountFrom=0  CountResetPort=off  CountLoadPort=off  CountEnbPort=on  CountDirPort=off  CountHitOutputPort=off  CountDataType=Unsigned  CountWordLen=16  CountFracLen=0  CountSampTime=1
  Delay : Delay  DelayLength=7  InitialCondition=0
  Delay1 : Delay  DelayLength=6  InitialCondition=0
  Delay2 : Delay  DelayLength=5  InitialCondition=0
  Delay3 : Delay  DelayLength=3  InitialCondition=0
  Delay4 : Delay  InitialCondition=0
  Delay5 : Delay  DelayLength=1  InitialCondition=0
  Delay6 : Delay  DelayLength=4  InitialCondition=0
  Rectangular QAM Modulator Baseband : commdigbbndam3/Rectangular QAM Modulator Baseband  M=256  InType=Integer  Enc=Gray  Mapping=[0:15]  PowType=Min. distance between symbols  MinDist=2  AvgPow=1  PeakPow=1  Ph=0  outDtype=double  outWordLen=16  outUDDataType=sfix(16)  outFracLenMode=Best precision  outFracLen=15  outDataTypeStr=double  outLastDataTypeStr=double
      settings: LibrarySourceBlock=|
      | commhdldigbbndam/Rectangular QAM
      | Modulator
      | Baseband
  data lookup : LookupNDDirect  NumberOfTableDimensions=1  Table=qam_params.tx_data_bits  DiagnosticForOutOfRangeInput=Error  SampleTime=1/qam_params.bitRate  TableDataTypeStr=boolean
  Out1 : Outport
  wires:
  data lookup/1 -> Bit Concat/8, Delay5/1, Delay4/1, Delay3/1, Delay6/1, Delay/1, Delay1/1, Delay2/1
  Delay5/1 -> Bit Concat/7
  Delay2/1 -> Bit Concat/3
  Delay3/1 -> Bit Concat/5
  Data Address Counter/1 -> data lookup/1
  Delay1/1 -> Bit Concat/2
  Bit Concat/1 -> Rectangular QAM Modulator Baseband/1
  Delay6/1 -> Bit Concat/4
  Delay/1 -> Bit Concat/1
  enb/1 -> Data Address Counter/1
  Delay4/1 -> Bit Concat/6
  Rectangular QAM Modulator Baseband/1 -> Out1/1  "QAMOutput"

== system Model0/multi-carrier system/Upconverter ==
  In : Inport
  Complex to Real-Imag : ComplexToRealImag  Output=Real
  Local Oscillator : dspsrcs4/Sine Wave  Amplitude=1  Frequency=200e6  Phase=0  SampleMode=Discrete  OutComplex=Complex  CompMethod=Trigonometric fcn  TableSize=Speed  SampleTime=(1e-6) /8  SamplesPerFrame=8  ResetState=Restart at time zero  OutputFrames=off  dataType=double  wordLen=16  udDataType=sfix(16)  fracBitsMode=Best precision  numFracBits=15  OutDataTypeStr=double  LastOutDataTypeStr=double
  Product : Product  RndMeth=Zero
  Out : Outport  VectorParamsAs1DForOutWhenUnconnected=off
  wires:
  Complex to Real-Imag/1 -> Out/1
  Product/1 -> Complex to Real-Imag/1
  Local Oscillator/1 -> Product/2
  In/1 -> Product/1

== system Model0/multi-carrier system/Upconverter1 ==
  In : Inport
  Complex to Real-Imag : ComplexToRealImag  Output=Real
  Local Oscillator : dspsrcs4/Sine Wave  Amplitude=1  Frequency=400e6  Phase=0  SampleMode=Discrete  OutComplex=Complex  CompMethod=Trigonometric fcn  TableSize=Speed  SampleTime=(1e-6) /8  SamplesPerFrame=8  ResetState=Restart at time zero  OutputFrames=off  dataType=double  wordLen=16  udDataType=sfix(16)  fracBitsMode=Best precision  numFracBits=15  OutDataTypeStr=double  LastOutDataTypeStr=double
  Product : Product  RndMeth=Zero
  Out : Outport  VectorParamsAs1DForOutWhenUnconnected=off
  wires:
  Complex to Real-Imag/1 -> Out/1
  Product/1 -> Complex to Real-Imag/1
  Local Oscillator/1 -> Product/2
  In/1 -> Product/1

== system Model0/multi-carrier system/Upconverter2 ==
  In : Inport
  Complex to Real-Imag : ComplexToRealImag  Output=Real
  Local Oscillator : dspsrcs4/Sine Wave  Amplitude=1  Frequency=600e6  Phase=0  SampleMode=Discrete  OutComplex=Complex  CompMethod=Trigonometric fcn  TableSize=Speed  SampleTime=(1e-6) /8  SamplesPerFrame=8  ResetState=Restart at time zero  OutputFrames=off  dataType=double  wordLen=16  udDataType=sfix(16)  fracBitsMode=Best precision  numFracBits=15  OutDataTypeStr=double  LastOutDataTypeStr=double
  Product : Product  RndMeth=Zero
  Out : Outport  VectorParamsAs1DForOutWhenUnconnected=off
  wires:
  Complex to Real-Imag/1 -> Out/1
  Product/1 -> Complex to Real-Imag/1
  Local Oscillator/1 -> Product/2
  In/1 -> Product/1

== system Model0/multi-carrier system/Upconverter3 ==
  In : Inport
  Complex to Real-Imag : ComplexToRealImag  Output=Real
  Local Oscillator : dspsrcs4/Sine Wave  Amplitude=1  Frequency=800e6  Phase=0  SampleMode=Discrete  OutComplex=Complex  CompMethod=Trigonometric fcn  TableSize=Speed  SampleTime=(1e-6) /8  SamplesPerFrame=8  ResetState=Restart at time zero  OutputFrames=off  dataType=double  wordLen=16  udDataType=sfix(16)  fracBitsMode=Best precision  numFracBits=15  OutDataTypeStr=double  LastOutDataTypeStr=double
  Product : Product  RndMeth=Zero
  Out : Outport  VectorParamsAs1DForOutWhenUnconnected=off
  wires:
  Complex to Real-Imag/1 -> Out/1
  Product/1 -> Complex to Real-Imag/1
  Local Oscillator/1 -> Product/2
  In/1 -> Product/1

== system Model0/multi-carrier system/Upconverter4 ==
  In : Inport
  Complex to Real-Imag : ComplexToRealImag  Output=Real
  Local Oscillator : dspsrcs4/Sine Wave  Amplitude=1  Frequency=1e9  Phase=0  SampleMode=Discrete  OutComplex=Complex  CompMethod=Trigonometric fcn  TableSize=Speed  SampleTime=(1e-6) /8  SamplesPerFrame=8  ResetState=Restart at time zero  OutputFrames=off  dataType=double  wordLen=16  udDataType=sfix(16)  fracBitsMode=Best precision  numFracBits=15  OutDataTypeStr=double  LastOutDataTypeStr=double
  Product : Product  RndMeth=Zero
  Out : Outport  VectorParamsAs1DForOutWhenUnconnected=off
  wires:
  Complex to Real-Imag/1 -> Out/1
  Product/1 -> Complex to Real-Imag/1
  Local Oscillator/1 -> Product/2
  In/1 -> Product/1
